simulink model "pin"  (R2022b)
settings: Solver=FixedStepAuto  StartTime=0.0  StopTime=10.0  RelTol=1e-3  EnableMultiTasking=on
libraries: raspberrypiBasiclib x12
settings Model: SimulationMode=external  Creator=richa  LastModifiedBy=richa
settings SolverCC: PositivePriorityOrder=on
settings OptimizationCC: EnhancedBackFolding=on  PassReuseOutputArgsAs=Individual arguments  ZeroExternalMemoryAtStartup=off  ZeroInternalMemoryAtStartup=off  MaxStackSize=64  OptimizeBlockOrder=speed  DifferentSizesBufferReuse=on  OptimizationCustomize=off  EfficientTunableParamExpr=on
settings DebuggingCC: ParameterTunabilityLossMsg=error
settings HardwareCC: ProdBitPerPointer=32  ProdBitPerSizeT=32  ProdBitPerPtrDiffT=32  ProdLargestAtomicInteger=Long  ProdLargestAtomicFloat=Double  ProdWordSize=32  ProdLongLongMode=on  ProdHWDeviceType=ARM Compatible->ARM Cortex  UseEmbeddedCoderFeatures=off  UseSimulinkCoderFeatures=off
settings RTWCC: Description=Embedded Coder  SystemTargetFile=ert.tlc  HardwareBoard=Raspberry Pi  TLCOptions="-aInlineSetEventsForThisBaseRateFcn=TLC_FALSE -aSuppressMultiTaskScheduler=TLC_FALSE  -aRateBasedStepFcn=0"  TemplateMakefile=ert_default_tmf  Toolchain=GNU GCC Embedded Linux  BuildConfiguration=Faster Runs
settings CodeAppCC: ForceParamTrailComments=on  IgnoreCustomStorageClasses=off  OperatorAnnotations=on  SimulinkDataObjDesc=on  SFDataObjDesc=on  MangleLength=10  InsertBlockDesc=on
settings ERTTargetCC: SupportNonInlinedSFcns=on  SupportVariableSizeSignals=on  ExtModeTransport=2  ExtModeStaticAlloc=on  ExtModeMexFile=ext_xcp  ExtModeIntrfLevel=Level2 - Open

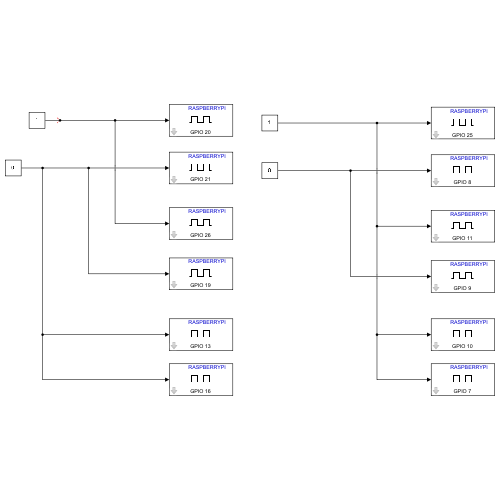
[thumbnail: Simulink's stored preview of the top-level diagram]
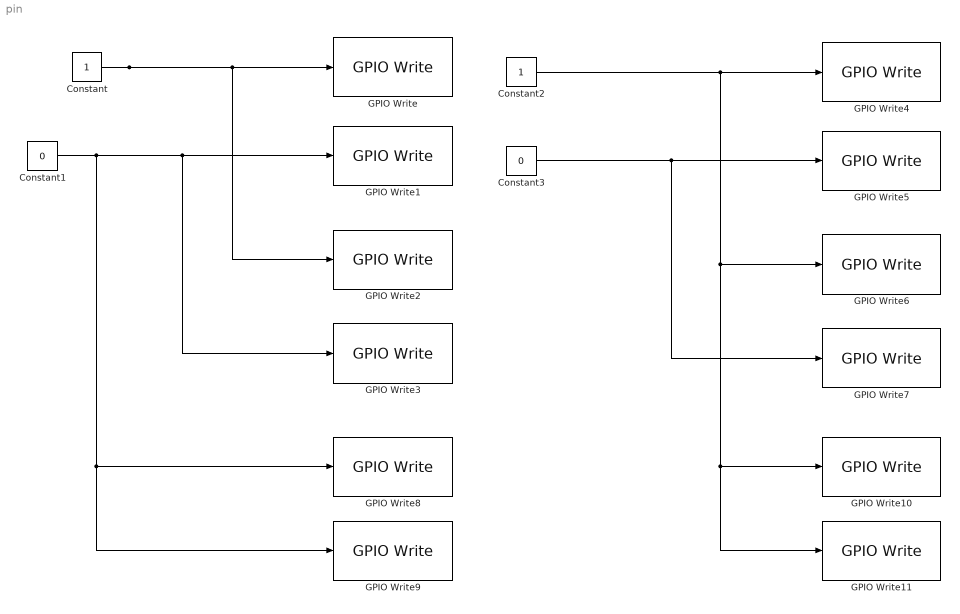
== system pin ==
  Constant : Constant
  Constant1 : Constant  Value=0
  Constant2 : Constant
  Constant3 : Constant  Value=0
  GPIO Write : raspberrypiBasiclib/GPIO Write  board=Pi 4 Model B  gpio=20  direction=Output  blockPlatform=Raspberry Pi
  GPIO Write1 : raspberrypiBasiclib/GPIO Write  board=Pi 4 Model B  gpio=21  direction=Output  blockPlatform=Raspberry Pi
  GPIO Write10 : raspberrypiBasiclib/GPIO Write  board=Pi 4 Model B  gpio=10  direction=Output  blockPlatform=Raspberry Pi
  GPIO Write11 : raspberrypiBasiclib/GPIO Write  board=Pi 4 Model B  gpio=7  direction=Output  blockPlatform=Raspberry Pi
  GPIO Write2 : raspberrypiBasiclib/GPIO Write  board=Pi 4 Model B  gpio=26  direction=Output  blockPlatform=Raspberry Pi
  GPIO Write3 : raspberrypiBasiclib/GPIO Write  board=Pi 4 Model B  gpio=19  direction=Output  blockPlatform=Raspberry Pi
  GPIO Write4 : raspberrypiBasiclib/GPIO Write  board=Pi 4 Model B  gpio=25  direction=Output  blockPlatform=Raspberry Pi
  GPIO Write5 : raspberrypiBasiclib/GPIO Write  board=Pi 4 Model B  gpio=8  direction=Output  blockPlatform=Raspberry Pi
  GPIO Write6 : raspberrypiBasiclib/GPIO Write  board=Pi 4 Model B  gpio=11  direction=Output  blockPlatform=Raspberry Pi
  GPIO Write7 : raspberrypiBasiclib/GPIO Write  board=Pi 4 Model B  gpio=9  direction=Output  blockPlatform=Raspberry Pi
  GPIO Write8 : raspberrypiBasiclib/GPIO Write  board=Pi 4 Model B  gpio=13  direction=Output  blockPlatform=Raspberry Pi
  GPIO Write9 : raspberrypiBasiclib/GPIO Write  board=Pi 4 Model B  gpio=16  direction=Output  blockPlatform=Raspberry Pi
  wires:
  Constant/1 -> GPIO Write2/1, GPIO Write/1
  Constant1/1 -> GPIO Write9/1, GPIO Write8/1, GPIO Write3/1, GPIO Write1/1
  Constant2/1 -> GPIO Write10/1, GPIO Write11/1, GPIO Write6/1, GPIO Write4/1
  Constant3/1 -> GPIO Write7/1, GPIO Write5/1
